simulink model "projemodel2"  (R2019a)
settings: Solver=VariableStepAuto  StartTime=0.0  StopTime=10.0  RelTol=1e-3
undefined symbols (not defined in the file or in its folder): Continuous, Time
libraries: ctrlSharedLib x3
settings Model: Creator=tr531  LastModifiedBy=tr531

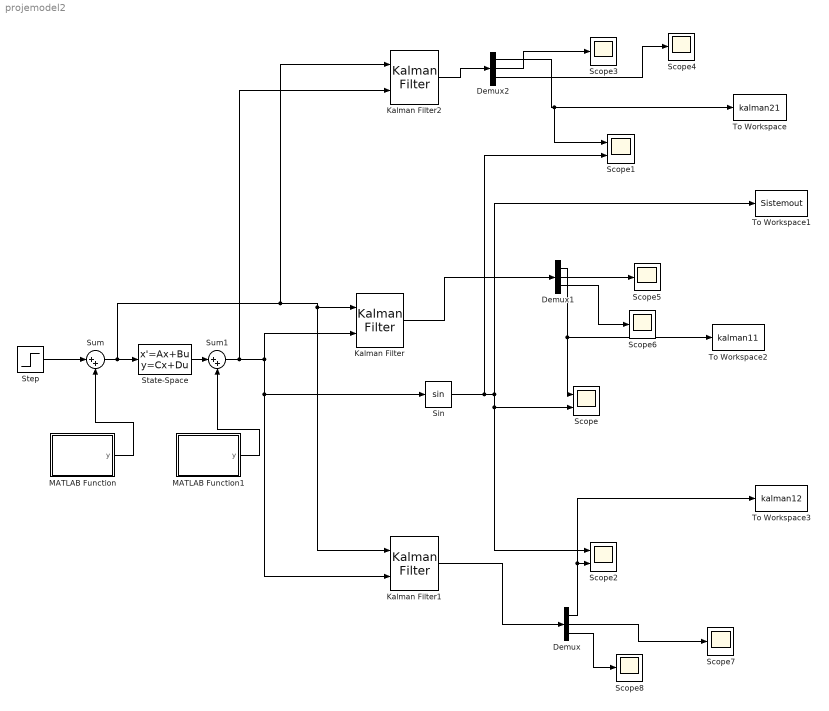
== system projemodel2 ==
  Demux : Demux  Outputs=3
  Demux1 : Demux  Outputs=3
  Demux2 : Demux  Outputs=3
  Kalman Filter : ctrlSharedLib/Kalman Filter  TimeDomain=Continuous-Time  UseCurrentEstimator=on  ModelSource=Individual A, B, C, D matrices  ModelSourceVariable=ss(0.95,1,1,0,1)  A=[1 1 0.5;0 1 1;0 0 1]  B=[0 ;0 ;0.125]  C=[1 0 0]  D=1  NumberOfStates=1  NumberOfInputs=1  NumberOfOutputs=1  InitialEstimateSource=Dialog  X0=0  P0=10  UseK=off  UseGH=off  NumberOfProcessNoiseInputs=1  G=1  TimeInvariantG=on  H=0  TimeInvariantH=on  Q=1  TimeInvariantQ=on  R=1  TimeInvariantR=on  N=0  TimeInvariantN=on  AddInputPort=on  AddEnablePort=off  OutputEstimatedY=off  OutputP=off  Ts=-1
      settings: SourceProductBaseCode=CT
  Kalman Filter1 : ctrlSharedLib/Kalman Filter  TimeDomain=Continuous-Time  UseCurrentEstimator=on  ModelSource=Individual A, B, C, D matrices  ModelSourceVariable=ss(0.95,1,1,0,1)  A=[1 1 0.5;0 1 1;0 0 1]  B=[0 ;0 ;0.125]  C=[1 0 0]  D=1  NumberOfStates=1  NumberOfInputs=1  NumberOfOutputs=1  InitialEstimateSource=Dialog  X0=0  P0=10  UseK=off  UseGH=off  NumberOfProcessNoiseInputs=1  G=1  TimeInvariantG=on  H=0  TimeInvariantH=on  Q=1  TimeInvariantQ=on  R=2  TimeInvariantR=on  N=0  TimeInvariantN=on  AddInputPort=on  AddEnablePort=off  OutputEstimatedY=off  OutputP=off  Ts=-1
      settings: SourceProductBaseCode=CT
  Kalman Filter2 : ctrlSharedLib/Kalman Filter  TimeDomain=Continuous-Time  UseCurrentEstimator=on  ModelSource=Individual A, B, C, D matrices  ModelSourceVariable=ss(0.95,1,1,0,1)  A=[1 1 0.5;0 1 1;0 0 1]  B=[0 ;0 ;0.125]  C=[1 0 0]  D=1  NumberOfStates=1  NumberOfInputs=1  NumberOfOutputs=1  InitialEstimateSource=Dialog  X0=0  P0=10  UseK=off  UseGH=off  NumberOfProcessNoiseInputs=1  G=1  TimeInvariantG=on  H=0  TimeInvariantH=on  Q=2  TimeInvariantQ=on  R=1  TimeInvariantR=on  N=0  TimeInvariantN=on  AddInputPort=on  AddEnablePort=off  OutputEstimatedY=off  OutputP=off  Ts=-1
      settings: SourceProductBaseCode=CT
  MATLAB Function : MATLAB Function  TreatAsAtomicUnit=on
  MATLAB Function1 : MATLAB Function  TreatAsAtomicUnit=on
  Scope : Scope  NumInputPorts=2
  Scope1 : Scope  NumInputPorts=2
  Scope2 : Scope  NumInputPorts=2
  Scope{3..8} (6 alike) : Scope
  Sin : Trigonometry
  State-Space : StateSpace  A=[1 1 1/2;0 1 1;0 0 1]  B=[0 ; 0; 1/80]  C=[1 0 0]  D=0  InitialCondition=0
  Step : Step  Time=0  After=0.00001  SampleTime=0
  Sum : Sum  Inputs=|++
  Sum1 : Sum  Inputs=|++
  To Workspace : ToWorkspace  VariableName=kalman21  SaveFormat=Timeseries  SampleTime=-1
  To Workspace1 : ToWorkspace  VariableName=Sistemout  SaveFormat=Timeseries  SampleTime=-1
  To Workspace2 : ToWorkspace  VariableName=kalman11  SaveFormat=Timeseries  SampleTime=-1
  To Workspace3 : ToWorkspace  VariableName=kalman12  SaveFormat=Timeseries  SampleTime=-1
  wires:
  Sum1/1 -> Kalman Filter2/2, Sin/1, Kalman Filter1/2, Kalman Filter/2
  MATLAB Function/1(y) -> Sum/2
  Step/1 -> Sum/1
  Sum/1 -> Kalman Filter2/1, Kalman Filter1/1, Kalman Filter/1, State-Space/1
  State-Space/1 -> Sum1/1
  MATLAB Function1/1(y) -> Sum1/2
  Sin/1 -> Scope1/2, Scope2/1, Scope/2, To Workspace1/1
  Kalman Filter1/1 -> Demux/1
  Demux/1 -> To Workspace3/1, Scope2/2
  Demux1/1 -> Scope/1, To Workspace2/1
  Kalman Filter/1 -> Demux1/1
  Kalman Filter2/1 -> Demux2/1
  Demux2/1 -> Scope1/1, To Workspace/1
  Demux2/2 -> Scope3/1
  Demux2/3 -> Scope4/1
  Demux1/2 -> Scope5/1
  Demux1/3 -> Scope6/1
  Demux/2 -> Scope7/1
  Demux/3 -> Scope8/1

== matlab function projemodel2/MATLAB Function1 ==
  data: y output
function y = fcn()
   cov_mat = 0.001;
   w = randn(1,1);
   w = cov_mat*w;
y = w;

== matlab function projemodel2/MATLAB Function ==
  data: y output
function y = fcn()
   cov_mat = 0.00001;
   w = randn(1,1);
   w = cov_mat*w;
y = w;
